simulink model "Task16"  (R2025a)
settings: Solver=VariableStepAuto  StartTime=0.0  StopTime=10.0  RelTol=1e-3
settings Model: Creator=LOQ  LastModifiedBy=LOQ

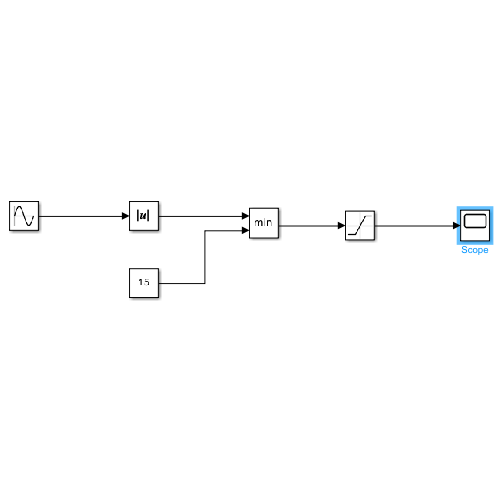
[thumbnail: Simulink's stored preview of the top-level diagram]
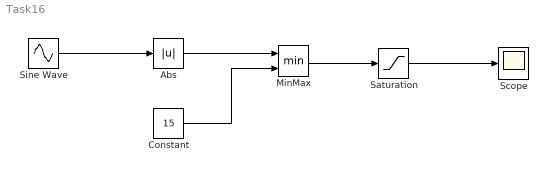
== system Task16 ==
  Abs : Abs  SaturateOnIntegerOverflow=off
  Constant : Constant  Value=15
  MinMax : MinMax  Inputs=2
  Saturation : Saturate  UpperLimit=10  LowerLimit=5
  Scope : Scope
      settings: ActiveDisplayYMinimum=4.375  ActiveDisplayYMaximum=10.625
  Sine Wave : Sin  Amplitude=20  SampleTime=0
  wires:
  Sine Wave/1 -> Abs/1
  Abs/1 -> MinMax/1
  Constant/1 -> MinMax/2
  MinMax/1 -> Saturation/1
  Saturation/1 -> Scope/1
